simulink model "dynamics_1d_function"  (R2018a)
settings: Solver=VariableStepAuto  StartTime=0.0  StopTime=10.0  RelTol=1e-3
settings Model: Creator=henry  LastModifiedBy=henry

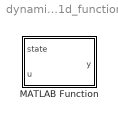
== system dynamics_1d_function ==
  MATLAB Function : MATLAB Function  TreatAsAtomicUnit=on

== matlab function dynamics_1d_function/MATLAB Function ==
  data: state input; u input; y output
function y = dynamics_1d(state, u)

l=.085;%m
lb=.075;%m
mb=.419;%kg
mw=.204;%kg
Ib=3.34*10^-3;
Iw=.57*10^-3;
Cb=1.02*10^-3;
Cw=.05*10^-3;
g=9.81;
k=25.1*10^-3;

theta_b=state(1);
theta_bdot=state(2);
theta_wdot=x(4);

f1=theta_bdot;
f2=((mb*lb+mw*l)*g*sin(theta_b)-k*u-Cb*theta_bdot+Cw*theta_wdot)/(Ib+mw*l^2);
f3=theta_wdot;
f4=(Ib+Iw+mw*l^2)*(k*u-Cw*theta_wdot)/(Iw*(Ib+mw*l^2))-((mb*lb+mw*l)*g*sin(theta_b)-Cb*theta_bdot)/(Ib+mw*l^2);

y = [f1;f2;f3;f4];

end
